simulink model "Lab2_1_sim"  (R2016b)
settings: Solver=VariableStepAuto  StartTime=0.0  StopTime=10.0  RelTol=1e-3  EnableMultiTasking=on
settings Model: Creator=Yash Bansod  LastModifiedBy=Yash Bansod
settings DataIOCC: LimitDataPoints=on
settings OptimizationCC: LifeSpan=inf
settings DebuggingCC: AllowSymbolicDim=off  SFUnexpectedBacktrackingDiag=warning  SFNoUnconditionalDefaultTransitionDiag=warning  SFExecutionAtInitializationDiag=none
settings ModelReferenceCC: PropagateSignalLabelsOutOfModel=off
settings GRTTargetCC: TargetLangStandard=C89/C90 (ANSI)
settings ConfigComp: CovMetricSettings=dw  CovHtmlReporting=on  CovSaveCumulativeToWorkspaceVar=on  CovSaveSingleToWorkspaceVar=on  CovExternalEMLEnable=off

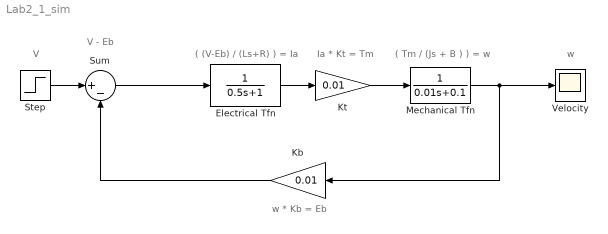
== system Lab2_1_sim ==
  note: w
  note: V - Eb
  note: V
  note: w * Kb = Eb
  note: ( Tm / (Js + B ) ) = w
  note: Ia * Kt = Tm
  note: ( (V-Eb) / (Ls+R) ) = Ia
  Electrical Tfn : TransferFcn  Denominator=[0.5 1]
  Kb : Gain  Gain=0.01
  Kt : Gain  Gain=0.01
  "Mechanical Tfn " : TransferFcn  Denominator=[0.01 0.1]
  Step : Step  After=220  SampleTime=0
  Sum : Sum  Inputs=|+-
  Velocity : Scope
  wires:
  Sum/1 -> Electrical Tfn/1
  Step/1 -> Sum/1
  Electrical Tfn/1 -> Kt/1
  Kt/1 -> "Mechanical Tfn "/1
  "Mechanical Tfn "/1 -> Velocity/1, Kb/1
  Kb/1 -> Sum/2
